simulink model "brain_tumor_baseline"  (R2024a)
settings: Solver=VariableStepAuto  StartTime=0.0  StopTime=2.5  RelTol=1e-3
settings Model: Creator=samad  LastModifiedBy=samad

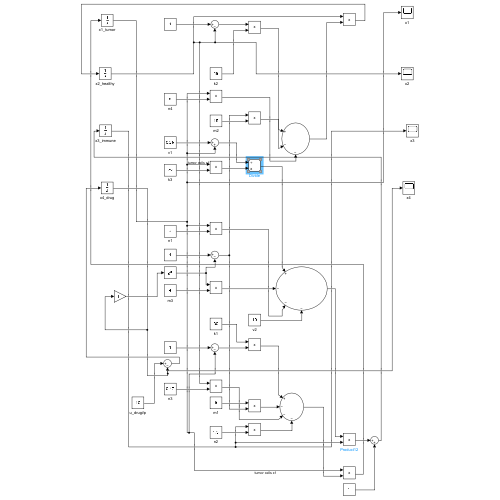
[thumbnail: Simulink's stored preview of the top-level diagram]
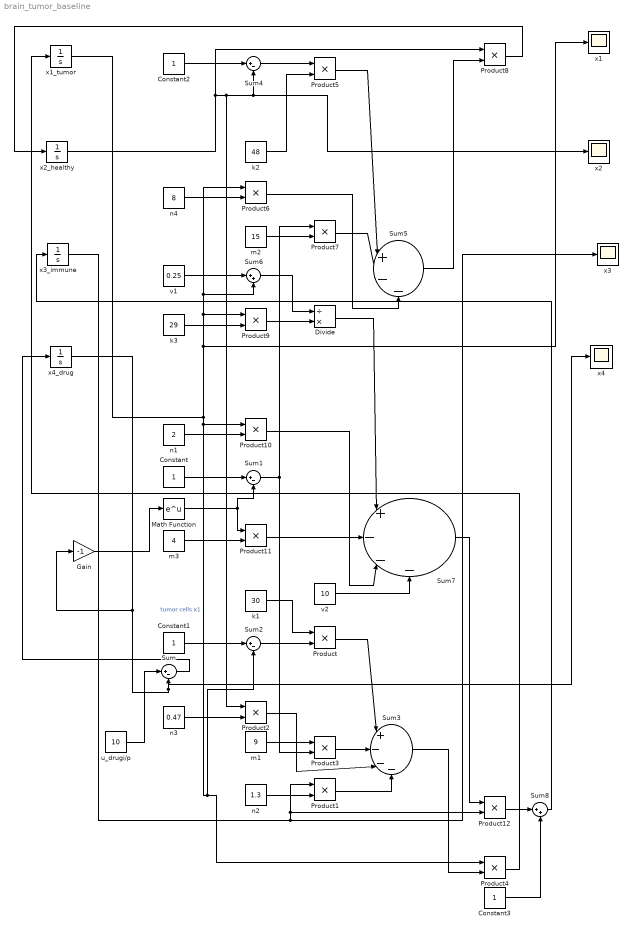
== system brain_tumor_baseline ==
  Constant{,1..3} (4 alike) : Constant
  Divide : Product  Inputs=/*
  Gain : Gain  Gain=-1
  Math Function : Math
  Product{,1..12} (13 alike) : Product
  Sum{,1..2,4} (4 alike) : Sum  Inputs=|+-
  Sum3 : Sum  Inputs=|+---
  Sum5 : Sum  Inputs=|+--
  Sum6 : Sum  Inputs=|++
  Sum7 : Sum  Inputs=|+---
  Sum8 : Sum  Inputs=|++
  k1 : Constant  Value=30
  k2 : Constant  Value=48
  k3 : Constant  Value=29
  m1 : Constant  Value=9
  m2 : Constant  Value=15
  m3 : Constant  Value=4
  n1 : Constant  Value=2
  n2 : Constant  Value=1.3
  n3 : Constant  Value=0.47
  n4 : Constant  Value=8
  u_drugi/p : Constant  Value=10
  v1 : Constant  Value=0.25
  v2 : Constant  Value=10
  x{1..4} (4 alike) : Scope
  x1_tumor : Integrator  InitialCondition=2.5
  x2_healthy : Integrator  InitialCondition=0.25
  x3_immune : Integrator  InitialCondition=1.55
  x4_drug : Integrator
  wires:
  Sum7/1 -> Product12/1
  x2_healthy/1 -> x2/1, Sum4/2, Product2/1, Product8/1
  x4_drug/1 -> x4/1, Sum/2, Gain/1
  m1/1 -> Product3/1
  n3/1 -> Product2/2
  u_drugi/p/1 -> Sum/1
  n1/1 -> Product10/2
  n2/1 -> Product1/2
  m2/1 -> Product7/2
  n4/1 -> Product6/2
  k3/1 -> Product9/2
  Divide/1 -> Sum7/1
  Constant/1 -> Sum1/1
  Constant2/1 -> Sum4/1
  Product11/1 -> Sum7/2
  v1/1 -> Sum6/1
  Product1/1 -> Sum3/4
  Product/1 -> Sum3/1
  Product10/1 -> Sum7/3
  m3/1 -> Product11/2
  Math Function/1 -> Sum1/2, Product11/1
  Constant1/1 -> Sum2/1
  Sum3/1 -> Product4/2
  Sum2/1 -> Product/2
  Sum1/1 -> Product3/2, Product7/1
  Sum/1 -> x4_drug/1
  x1_tumor/1 -> Sum2/2, Product4/1, Product10/1, Sum6/2, Product6/1, Product9/1, x1/1  "tumor cells x1"
  Sum5/1 -> Product8/2
  Sum4/1 -> Product5/1
  Sum6/1 -> Divide/1
  k2/1 -> Product5/2
  Product8/1 -> x2_healthy/1
  Product7/1 -> Sum5/2
  Product9/1 -> Divide/2
  Product6/1 -> Sum5/3
  k1/1 -> Product/1
  Product4/1 -> x1_tumor/1
  Product3/1 -> Sum3/2
  Product5/1 -> Sum5/1
  Product2/1 -> Sum3/3
  x3_immune/1 -> Product12/2, Product1/1, x3/1
  v2/1 -> Sum7/4
  Product12/1 -> Sum8/1
  Constant3/1 -> Sum8/2
  Sum8/1 -> x3_immune/1
  Gain/1 -> Math Function/1
